simulink model "Symulacja"  (R2021b)
settings: Solver=VariableStepAuto  StartTime=0.0  StopTime=200  RelTol=1e-3
values from neighbouring files (symbols this model uses):
  K = 3    [ModiProjekt1.m]
  T = 1    [ModiProjekt1.m]
  T1 = 12    [ModiProjekt1.m]
  T2 = 5    [ModiProjekt1.m]
  Tp1 = 1.5    [ModiProjekt1.m]
  Tp2 = 6    [ModiProjekt1.m]
settings Model: Creator=Adam  LastModifiedBy=Adam

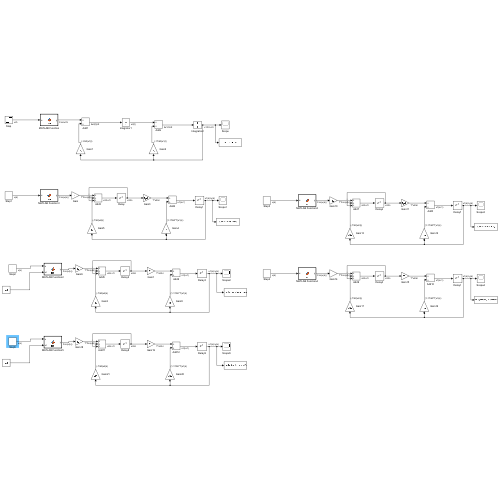
[thumbnail: Simulink's stored preview of the top-level diagram]
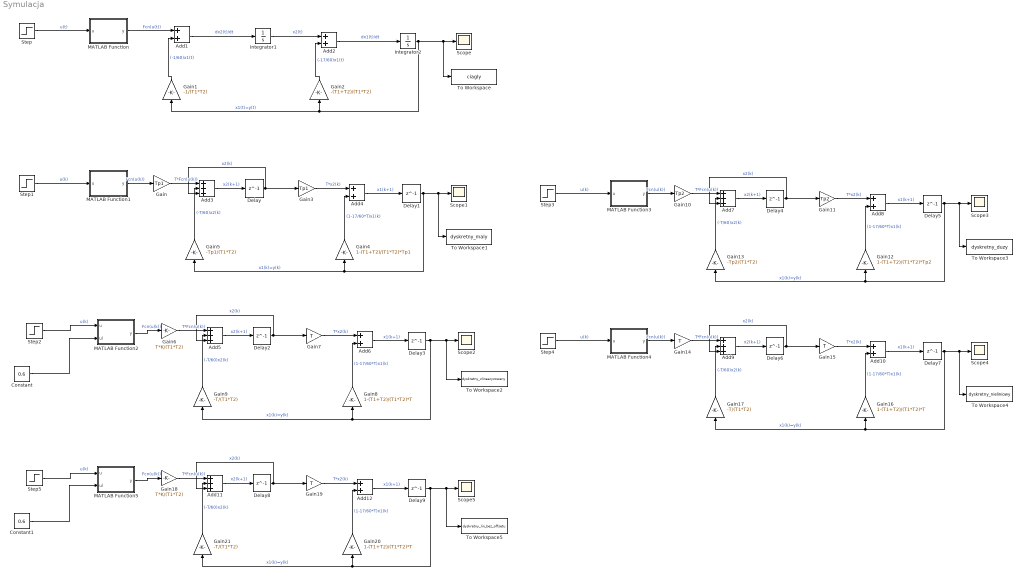
== system Symulacja ==
  Add{1..2,4,6,8,10,12} (7 alike) : Sum
  Add{3,5,7,9,11} (5 alike) : Sum  Inputs=+++
  Constant : Constant  Value=0.6
  Constant1 : Constant  Value=0.6
  Delay : Delay  DelayLength=1  InitialCondition=0  SampleTime=Tp1
  Delay1 : Delay  DelayLength=1  InitialCondition=0  SampleTime=Tp1
  Delay{2..3,6..9} (6 alike) : Delay  DelayLength=1  InitialCondition=0  SampleTime=T
  Delay4 : Delay  DelayLength=1  InitialCondition=0  SampleTime=Tp2
  Delay5 : Delay  DelayLength=1  InitialCondition=0  SampleTime=Tp2
  Gain : Gain  Gain=Tp1
  Gain1 : Gain  Gain=-1/(T1*T2)
  Gain10 : Gain  Gain=Tp2
  Gain11 : Gain  Gain=Tp2
  Gain12 : Gain  Gain=1-(T1+T2)/(T1*T2)*Tp2
  Gain13 : Gain  Gain=-Tp2/(T1*T2)
  Gain{7,14..15,19} (4 alike) : Gain  Gain=T
  Gain16 : Gain  Gain=1-(T1+T2)/(T1*T2)*T
  Gain17 : Gain  Gain=-T/(T1*T2)
  Gain18 : Gain  Gain=T*K/(T1*T2)
  Gain2 : Gain  Gain=-(T1+T2)/(T1*T2)
  Gain20 : Gain  Gain=1-(T1+T2)/(T1*T2)*T
  Gain21 : Gain  Gain=-T/(T1*T2)
  Gain3 : Gain  Gain=Tp1
  Gain4 : Gain  Gain=1-(T1+T2)/(T1*T2)*Tp1
  Gain5 : Gain  Gain=-Tp1/(T1*T2)
  Gain6 : Gain  Gain=T*K/(T1*T2)
  Gain8 : Gain  Gain=1-(T1+T2)/(T1*T2)*T
  Gain9 : Gain  Gain=-T/(T1*T2)
  Integrator1 : Integrator
  Integrator2 : Integrator
  MATLAB Function : MATLAB Function  TreatAsAtomicUnit=on
  MATLAB Function1 : MATLAB Function  TreatAsAtomicUnit=on
  MATLAB Function2 : MATLAB Function  TreatAsAtomicUnit=on
  MATLAB Function3 : MATLAB Function  TreatAsAtomicUnit=on
  MATLAB Function4 : MATLAB Function  TreatAsAtomicUnit=on
  MATLAB Function5 : MATLAB Function  TreatAsAtomicUnit=on
  Scope{,1..5} (6 alike) : Scope
  Step{,1..5} (6 alike) : Step  Time=10  SampleTime=0
  To Workspace : ToWorkspace  VariableName=ciagly  SaveFormat=Structure With Time  SampleTime=-1
  To Workspace1 : ToWorkspace  VariableName=dyskretny_maly  SaveFormat=Structure With Time  SampleTime=-1
  To Workspace2 : ToWorkspace  VariableName=dyskretny_zlinearyzowany  SaveFormat=Structure With Time  SampleTime=-1
  To Workspace3 : ToWorkspace  VariableName=dyskretny_duzy  SaveFormat=Structure With Time  SampleTime=-1
  To Workspace4 : ToWorkspace  VariableName=dyskretny_nieliniowy  SaveFormat=Structure With Time  SampleTime=-1
  To Workspace5 : ToWorkspace  VariableName=dyskretny_lin_bez_offsetu  SaveFormat=Structure With Time  SampleTime=-1
  wires:
  MATLAB Function/1(y) -> Add1/1  "Fcn(u(t))"
  Add1/1 -> Integrator1/1  "dx2(t)/dt"
  Integrator1/1 -> Add2/1  "x2(t)"
  Add2/1 -> Integrator2/1  "dx1(t)/dt"
  Integrator2/1 -> Gain1/1, Gain2/1, To Workspace/1, Scope/1  "x1(t)=y(t)"
  Gain1/1 -> Add1/2  "(-1/60)x1(t)"
  Gain2/1 -> Add2/2  "(-17/60)x1(t)"
  Step/1 -> MATLAB Function/1(u)  "u(t)"
  Step1/1 -> MATLAB Function1/1(u)  "u(k)"
  MATLAB Function1/1(y) -> Gain/1  "Fcn(u(k))"
  Gain/1 -> Add3/1  "T*Fcn(u(k))"
  Add3/1 -> Delay/1  "x2(k+1)"
  Delay/1 -> Add3/3, Gain3/1  "x2(k)"
  Gain3/1 -> Add4/1  "T*x2(k)"
  Add4/1 -> Delay1/1  "x1(k+1)"
  Delay1/1 -> Gain5/1, Gain4/1, To Workspace1/1, Scope1/1  "x1(k)=y(k)"
  Gain4/1 -> Add4/2  "(1-17/60*T)x1(k)"
  Gain5/1 -> Add3/2  "(-T/60)x2(k)"
  Gain9/1 -> Add5/2  "(-T/60)x2(k)"
  Delay2/1 -> Add5/3, Gain7/1  "x2(k)"
  Delay3/1 -> Gain9/1, Gain8/1, To Workspace2/1, Scope2/1  "x1(k)=y(k)"
  MATLAB Function2/1(y) -> Gain6/1  "Fcn(u(k))"
  Gain6/1 -> Add5/1  "T*Fcn(u(k))"
  Add5/1 -> Delay2/1  "x2(k+1)"
  Gain8/1 -> Add6/2  "(1-17/60*T)x1(k)"
  Gain7/1 -> Add6/1  "T*x2(k)"
  Add6/1 -> Delay3/1  "x1(k+1)"
  Step2/1 -> MATLAB Function2/1(u)  "u(k)"
  Constant/1 -> MATLAB Function2/2(ul)
  Add8/1 -> Delay5/1  "x1(k+1)"
  Delay5/1 -> Gain13/1, Gain12/1, To Workspace3/1, Scope3/1  "x1(k)=y(k)"
  Gain12/1 -> Add8/2  "(1-17/60*T)x1(k)"
  MATLAB Function3/1(y) -> Gain10/1  "Fcn(u(k))"
  Add7/1 -> Delay4/1  "x2(k+1)"
  Gain13/1 -> Add7/2  "(-T/60)x2(k)"
  Gain10/1 -> Add7/1  "T*Fcn(u(k))"
  Delay4/1 -> Add7/3, Gain11/1  "x2(k)"
  Step3/1 -> MATLAB Function3/1(u)  "u(k)"
  Gain11/1 -> Add8/1  "T*x2(k)"
  Add10/1 -> Delay7/1  "x1(k+1)"
  Delay7/1 -> Gain17/1, Gain16/1, To Workspace4/1, Scope4/1  "x1(k)=y(k)"
  Gain16/1 -> Add10/2  "(1-17/60*T)x1(k)"
  MATLAB Function4/1(y) -> Gain14/1  "Fcn(u(k))"
  Add9/1 -> Delay6/1  "x2(k+1)"
  Gain17/1 -> Add9/2  "(-T/60)x2(k)"
  Gain14/1 -> Add9/1  "T*Fcn(u(k))"
  Delay6/1 -> Add9/3, Gain15/1  "x2(k)"
  Step4/1 -> MATLAB Function4/1(u)  "u(k)"
  Gain15/1 -> Add10/1  "T*x2(k)"
  Constant1/1 -> MATLAB Function5/2(ul)
  Add11/1 -> Delay8/1  "x2(k+1)"
  Add12/1 -> Delay9/1  "x1(k+1)"
  Gain20/1 -> Add12/2  "(1-17/60*T)x1(k)"
  Step5/1 -> MATLAB Function5/1(u)  "u(k)"
  Gain21/1 -> Add11/2  "(-T/60)x2(k)"
  Delay9/1 -> Gain21/1, Gain20/1, To Workspace5/1, Scope5/1  "x1(k)=y(k)"
  Gain18/1 -> Add11/1  "T*Fcn(u(k))"
  Gain19/1 -> Add12/1  "T*x2(k)"
  Delay8/1 -> Add11/3, Gain19/1  "x2(k)"
  MATLAB Function5/1(y) -> Gain18/1  "Fcn(u(k))"

== matlab function Symulacja/MATLAB Function ==
  data: u input; y output
function y = fcn(u)
alfa1 = 0.6;
alfa2 = 1.35;
alfa3 = -0.57;
alfa4 = 0.53;
K = 3;
T1 = 12;
T2 = 5;
y = (K/(T1*T2))*(alfa1*u+alfa2*u^2+alfa3*u^3+alfa4*u^4);

== matlab function Symulacja/MATLAB Function2 ==
  data: u input; y output; ul input
function y = fcn(u,ul)
y = u*(0.6+2.7*ul-1.71*ul^2+2.12*ul^3)+(-1.35*ul^2+1.14*ul^3-1.59*ul^4);

== matlab function Symulacja/MATLAB Function3 ==
  data: u input; y output
function y = fcn(u)
alfa1 = 0.6;
alfa2 = 1.35;
alfa3 = -0.57;
alfa4 = 0.53;
K = 3;
T1 = 12;
T2 = 5;
y = (K/(T1*T2))*(alfa1*u+alfa2*u^2+alfa3*u^3+alfa4*u^4);

== matlab function Symulacja/MATLAB Function4 ==
  data: u input; y output
function y = fcn(u)
alfa1 = 0.6;
alfa2 = 1.35;
alfa3 = -0.57;
alfa4 = 0.53;
K = 3;
T1 = 12;
T2 = 5;
y = (K/(T1*T2))*(alfa1*u+alfa2*u^2+alfa3*u^3+alfa4*u^4);

== matlab function Symulacja/MATLAB Function5 ==
  data: u input; y output; ul input
function y = fcn(u,ul)
y = u*(0.6+2.7*ul-1.71*ul^2+2.12*ul^3);

== matlab function Symulacja/MATLAB Function1 ==
  data: u input; y output
function y = fcn(u)
alfa1 = 0.6;
alfa2 = 1.35;
alfa3 = -0.57;
alfa4 = 0.53;
K = 3;
T1 = 12;
T2 = 5;
y = (K/(T1*T2))*(alfa1*u+alfa2*u^2+alfa3*u^3+alfa4*u^4);
